simulink subsystem "Flight_Sensors"  (R2023b)
settings: Solver=VariableStepAuto  StartTime=0.0  StopTime=10.0  RelTol=1e-3
libraries: aerolibasang x1, aerolibatmos2 x1
settings Model: Creator=szdaniel  LastModifiedBy=USER

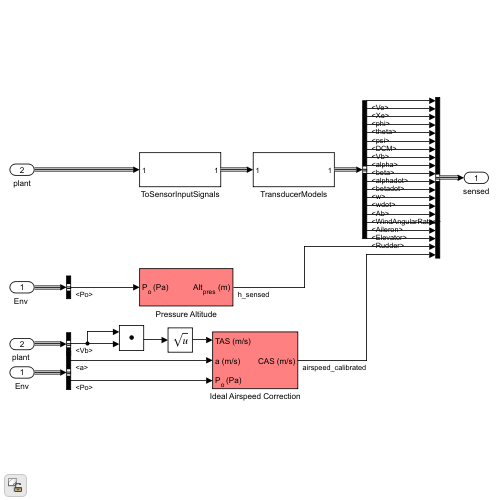
[thumbnail: Simulink's stored preview of the top-level diagram]
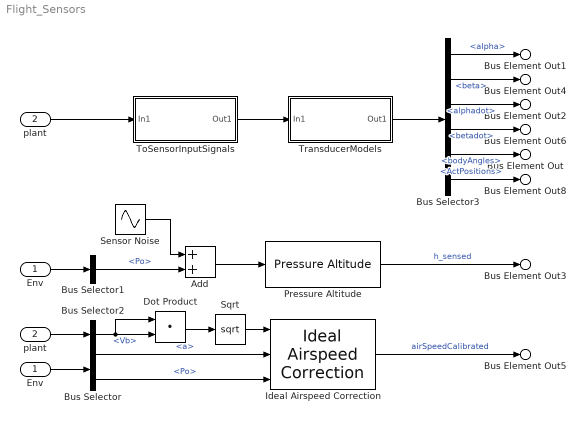
== system Flight_Sensors ==
  Env : Inport
  plant : Inport  Port=2  OutDataTypeStr=Bus: PlantDataBus
  Add : Sum
  Bus Selector : BusSelector  OutputSignals=a,Po
  Bus Selector1 : BusSelector  OutputSignals=Po
  Bus Selector2 : BusSelector  OutputSignals=Vb
  Bus Selector3 : BusSelector  OutputSignals=alpha,beta,alphadot,betadot,bodyAngles,ActPositions
  Dot Product : DotProduct  OutDataTypeStr=Inherit: Inherit via internal rule
  "Env " : InportShadow
  Ideal Airspeed Correction : aerolibasang/Ideal Airspeed Correction  units=Metric (MKS)  vel_in=TAS  vel_out_tas=CAS  vel_out_eas=CAS  vel_out_cas=TAS  method=Table Lookup  SubOnly=off  action=Error
  Pressure Altitude : aerolibatmos2/Pressure Altitude  units=Metric (MKS)  action=Warning
  Sensor Noise : Sin  Amplitude=10  Frequency=20*2*pi  SampleTime=0
  Sqrt : Sqrt
  ToSensorInputSignals : Subsystem
  TransducerModels : Subsystem
  "plant " : InportShadow  Port=2  OutDataTypeStr=Bus: PlantDataBus
  Bus Element Out8 : Outport  PortName=sensed  Element=ActPositions
  Bus Element Out : Outport  PortName=sensed  Element=bodyAngles
  Bus Element Out1 : Outport  PortName=sensed  Element=alpha
  Bus Element Out4 : Outport  PortName=sensed  Element=beta
  Bus Element Out2 : Outport  PortName=sensed  Element=alphadot
  Bus Element Out6 : Outport  PortName=sensed  Element=betadot
  Bus Element Out3 : Outport  PortName=sensed  Element=h_sensed
  Bus Element Out5 : Outport  PortName=sensed  Element=airSpeedCalibrated
  wires:
  ToSensorInputSignals/1(Out1) -> TransducerModels/1(In1)
  Env/1 -> Bus Selector/1
  TransducerModels/1(Out1) -> Bus Selector3/1
  plant/1 -> ToSensorInputSignals/1(In1)
  Bus Selector/1 -> Ideal Airspeed Correction/2  "<a>"
  Bus Selector/2 -> Ideal Airspeed Correction/3  "<Po>"
  Bus Selector1/1 -> Add/2  "<Po>"
  "Env "/1 -> Bus Selector1/1
  "plant "/1 -> Bus Selector2/1
  Dot Product/1 -> Sqrt/1
  Sqrt/1 -> Ideal Airspeed Correction/1
  Bus Selector2/1 -> Dot Product/1, Dot Product/2  "<Vb>"
  Bus Selector3/1 -> Bus Element Out1/1  "<alpha>"
  Bus Selector3/2 -> Bus Element Out4/1  "<beta>"
  Bus Selector3/3 -> Bus Element Out2/1  "<alphadot>"
  Bus Selector3/4 -> Bus Element Out6/1  "<betadot>"
  Bus Selector3/6 -> Bus Element Out8/1  "<ActPositions>"
  Pressure Altitude/1 -> Bus Element Out3/1  "h_sensed"
  Ideal Airspeed Correction/1 -> Bus Element Out5/1  "airSpeedCalibrated"
  Bus Selector3/5 -> Bus Element Out/1  "<bodyAngles>"
  Add/1 -> Pressure Altitude/1
  Sensor Noise/1 -> Add/1

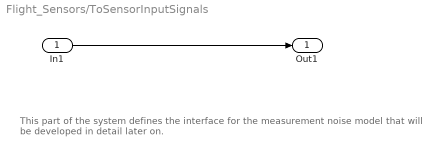
== system Flight_Sensors/ToSensorInputSignals ==
  note: This part of the system defines the interface for the measurement noise model that
      |  will be developed in detail later on.
  In1 : Inport
  Out1 : Outport  VectorParamsAs1DForOutWhenUnconnected=off
  wires:
  In1/1 -> Out1/1

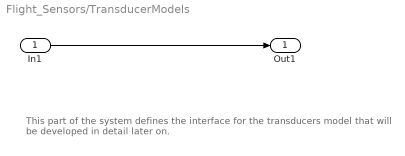
== system Flight_Sensors/TransducerModels ==
  note: This part of the system defines the interface for the transducers model that
      |  will be developed in detail later on.
  In1 : Inport
  Out1 : Outport  VectorParamsAs1DForOutWhenUnconnected=off
  wires:
  In1/1 -> Out1/1
